simulink model "check_stm32"  (R2020b)
settings: Solver=FixedStepDiscrete  StartTime=0.0  StopTime=inf  FixedStep=0.1  RelTol=1e-3
undefined symbols (not defined in the file or in its folder): Serial_Port, Standard_Devices
libraries: sldrtlib x2, simulink x1
settings Model: DataTypeOverride=Double  MinMaxOverflowLogging=ForceOff  Creator=Rahul Subramanian  LastModifiedBy=Rahul Subramanian

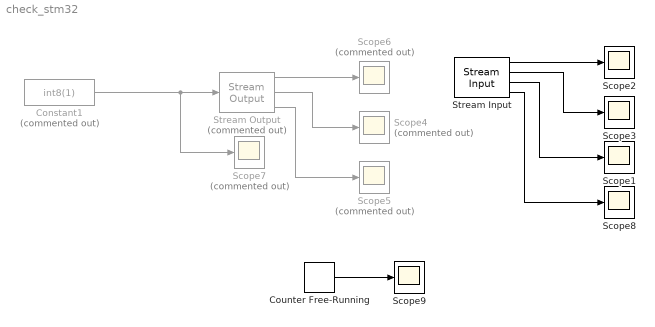
== system check_stm32 ==
  Constant1 : Constant  Commented=on  Value=int8(1)
  Counter Free-Running : simulink/Sources/Counter Free-Running  NumBits=4  tsamp=-1
  Scope{1..3,8..9} (5 alike) : Scope
  Scope{4..7} (4 alike) : Scope  Commented=on
  Stream Input : sldrtlib/Stream Input  SampleTime=0.1  MaxMissedTicks=inf  ShowMissedTicks=on  YieldWhenWaiting=off  DrvName=Standard_Devices/Serial_Port  DrvAddress=3  DrvOptions=[9600 8 0 0 0 0 0 1]  DataTypes='int8'  FormatString='%d'  Terminator={'\n'}  ShowReady=on  ShowError=on
      settings: AttributesFormatString=Serial Port [3]  SourceProductBaseCode=WT
  Stream Output : sldrtlib/Stream Output  Commented=on  SampleTime=0.1  MaxMissedTicks=inf  ShowMissedTicks=on  YieldWhenWaiting=off  DrvName=Standard_Devices/Serial_Port  DrvAddress=4  DrvOptions=[9600 8 0 0 0 0 0 0]  PortSizes=[1]  FormatString='%d\n'  ShowReady=on  ShowError=on  InitialValue=[]  FinalValue=[]
      settings: AttributesFormatString=Serial Port [4]  SourceProductBaseCode=WT
  wires:
  Stream Input/1 -> Scope2/1
  Stream Output/1 -> Scope6/1
  Stream Output/2 -> Scope4/1
  Stream Output/3 -> Scope5/1
  Constant1/1 -> Scope7/1, Stream Output/1
  Stream Input/2 -> Scope3/1
  Stream Input/3 -> Scope1/1
  Stream Input/4 -> Scope8/1
  Counter Free-Running/1 -> Scope9/1
